simulink model "targeting_subsystem"  (R2020a)
settings: Solver=VariableStepAuto  StartTime=0.0  StopTime=10.0  RelTol=1e-3
settings Model: Creator=Tamer  LastModifiedBy=Tamer

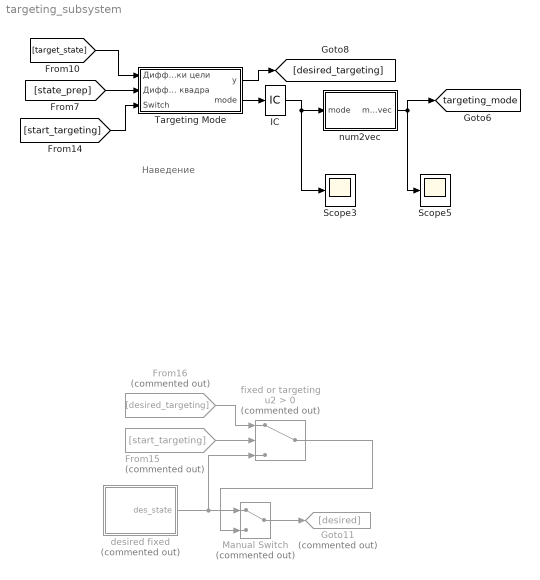
== system targeting_subsystem ==
  note: Наведение
  From15 : From  Commented=on  GotoTag=start_targeting
  From16 : From  Commented=on  GotoTag=desired_targeting
  Goto11 : Goto  Commented=on  GotoTag=desired
  IC : InitialCondition  Value=0
  Manual Switch : ManualSwitch  Commented=on
  Scope3 : Scope
  Scope5 : Scope
  Targeting Mode : Subsystem
  desired fixed : MATLAB Function  Commented=on  TreatAsAtomicUnit=on
  fixed or targeting : Switch  Commented=on  Criteria=u2 > Threshold
  num2vec : MATLAB Function  TreatAsAtomicUnit=on
  tag scope: targeting_mode=global
  wires:
  IC/1 -> num2vec/1(mode), Scope3/1
  num2vec/1(mode_vec) -> [targeting_mode], Scope5/1
  Targeting Mode/1(y) -> [desired_targeting]
  [target_state] -> Targeting Mode/1("Диффурочки цели ")
  Targeting Mode/2(mode) -> IC/1
  [start_targeting] -> Targeting Mode/3(Switch)
  [state_prep] -> Targeting Mode/2(Диффурочки квадра)
  fixed or targeting/1 -> Manual Switch/2
  From15/1 -> fixed or targeting/2
  desired fixed/1(des_state) -> fixed or targeting/3, Manual Switch/1
  From16/1 -> fixed or targeting/1
  Manual Switch/1 -> Goto11/1

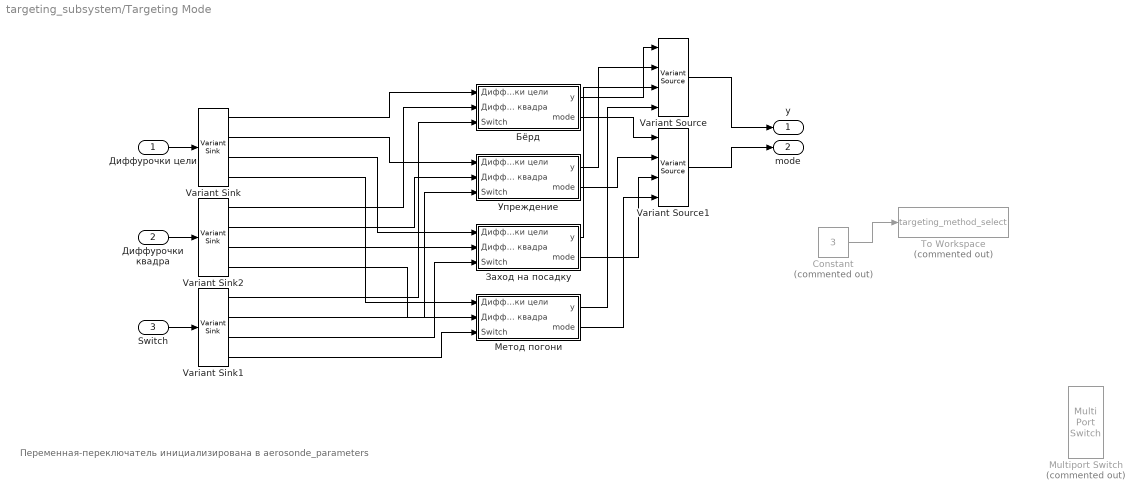
== system targeting_subsystem/Targeting Mode ==
  note: Переменная-переключатель инициализирована в aerosonde_parameters
  "Диффурочки цели " : Inport
  Диффурочки квадра : Inport  Port=2
  Switch : Inport  Port=3
  Constant : Constant  Commented=on  Value=3
  Multiport Switch : MultiPortSwitch  Commented=on  Inputs=4
  To Workspace : ToWorkspace  Commented=on  VariableName=targeting_method_select  SaveFormat=Timeseries  SampleTime=-1
  Variant Sink : VariantSink
  Variant Sink1 : VariantSink
  Variant Sink2 : VariantSink
  Variant Source : VariantSource
  Variant Source1 : VariantSource
  Бёрд : Subsystem
  Заход на посадку : Subsystem
  Метод погони : Subsystem
  Упреждение : Subsystem
  y : Outport
  mode : Outport  Port=2
  wires:
  Упреждение/1(y) -> Variant Source/2
  Упреждение/2(mode) -> Variant Source1/2
  Бёрд/2(mode) -> Variant Source1/1
  Бёрд/1(y) -> Variant Source/1
  Constant/1 -> To Workspace/1
  Заход на посадку/2(mode) -> Variant Source1/3
  Variant Source/1 -> y/1
  Variant Source1/1 -> mode/1
  Метод погони/1(y) -> Variant Source/4
  Метод погони/2(mode) -> Variant Source1/4
  "Диффурочки цели "/1 -> Variant Sink/1
  Диффурочки квадра/1 -> Variant Sink2/1
  Switch/1 -> Variant Sink1/1
  Variant Sink/1 -> Бёрд/1("Диффурочки цели ")
  Variant Sink/2 -> Упреждение/1("Диффурочки цели ")
  Variant Sink/3 -> Заход на посадку/1("Диффурочки цели ")
  Variant Sink/4 -> Метод погони/1("Диффурочки цели ")
  Variant Sink2/1 -> Бёрд/2(Диффурочки квадра)
  Variant Sink2/2 -> Упреждение/2(Диффурочки квадра)
  Variant Sink2/3 -> Заход на посадку/2(Диффурочки квадра)
  Variant Sink2/4 -> Метод погони/2(Диффурочки квадра)
  Variant Sink1/1 -> Бёрд/3(Switch)
  Variant Sink1/2 -> Упреждение/3(Switch)
  Variant Sink1/3 -> Заход на посадку/3(Switch)
  Variant Sink1/4 -> Метод погони/3(Switch)
  Заход на посадку/1(y) -> Variant Source/3

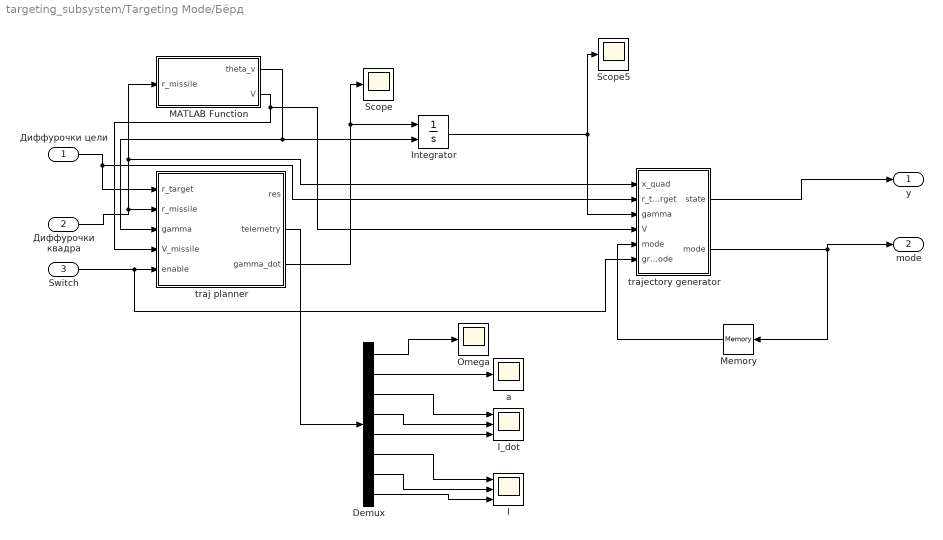
== system targeting_subsystem/Targeting Mode/Бёрд ==
  "Диффурочки цели " : Inport
  Диффурочки квадра : Inport  Port=2
  Switch : Inport  Port=3
  Demux : Demux  Outputs=8
  Integrator : Integrator  InitialConditionSource=external
  MATLAB Function : MATLAB Function  TreatAsAtomicUnit=on
  Memory : Memory
  Omega : Scope
  Scope : Scope
  Scope5 : Scope
  a : Scope
  l : Scope  NumInputPorts=3
  l_dot : Scope  NumInputPorts=3
  traj planner : MATLAB Function  TreatAsAtomicUnit=on
  trajectory generator : MATLAB Function  TreatAsAtomicUnit=on
  y : Outport
  mode : Outport  Port=2
  wires:
  "Диффурочки цели "/1 -> traj planner/1(r_target), trajectory generator/2(r_target)
  trajectory generator/1(state) -> y/1
  Диффурочки квадра/1 -> MATLAB Function/1(r_missile), trajectory generator/1(x_quad), traj planner/2(r_missile)
  MATLAB Function/1(theta_v) -> Integrator/2, traj planner/3(gamma)
  MATLAB Function/2(V) -> traj planner/4(V_missile), trajectory generator/4(V)
  traj planner/3(gamma_dot) -> Scope/1, Integrator/1
  Integrator/1 -> trajectory generator/3(gamma), Scope5/1
  trajectory generator/2(mode) -> mode/1, Memory/1
  Memory/1 -> trajectory generator/5("mode ")
  Switch/1 -> trajectory generator/6(grand_mode), traj planner/5(enable)
  traj planner/2(telemetry) -> Demux/1
  Demux/1 -> Omega/1
  Demux/2 -> a/1
  Demux/3 -> l_dot/1
  Demux/4 -> l_dot/2
  Demux/5 -> l_dot/3
  Demux/6 -> l/1
  Demux/7 -> l/2
  Demux/8 -> l/3

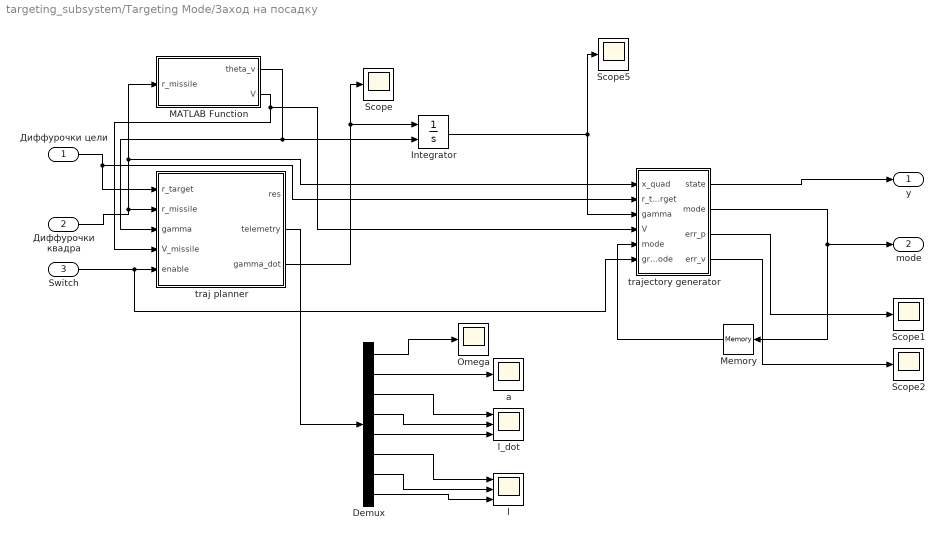
== system targeting_subsystem/Targeting Mode/Заход на посадку ==
  "Диффурочки цели " : Inport
  Диффурочки квадра : Inport  Port=2
  Switch : Inport  Port=3
  Demux : Demux  Outputs=8
  Integrator : Integrator  InitialConditionSource=external
  MATLAB Function : MATLAB Function  TreatAsAtomicUnit=on
  Memory : Memory
  Omega : Scope
  Scope{,1..2,5} (4 alike) : Scope
  a : Scope
  l : Scope  NumInputPorts=3
  l_dot : Scope  NumInputPorts=3
  traj planner : MATLAB Function  TreatAsAtomicUnit=on
  trajectory generator : MATLAB Function  TreatAsAtomicUnit=on
  y : Outport
  mode : Outport  Port=2
  wires:
  "Диффурочки цели "/1 -> traj planner/1(r_target), trajectory generator/2(r_target)
  trajectory generator/1(state) -> y/1
  Диффурочки квадра/1 -> MATLAB Function/1(r_missile), trajectory generator/1(x_quad), traj planner/2(r_missile)
  MATLAB Function/1(theta_v) -> Integrator/2, traj planner/3(gamma)
  MATLAB Function/2(V) -> traj planner/4(V_missile), trajectory generator/4(V)
  traj planner/3(gamma_dot) -> Scope/1, Integrator/1
  Integrator/1 -> trajectory generator/3(gamma), Scope5/1
  trajectory generator/2(mode) -> Memory/1, mode/1
  Memory/1 -> trajectory generator/5("mode ")
  Switch/1 -> trajectory generator/6(grand_mode), traj planner/5(enable)
  traj planner/2(telemetry) -> Demux/1
  Demux/1 -> Omega/1
  Demux/2 -> a/1
  Demux/3 -> l_dot/1
  Demux/4 -> l_dot/2
  Demux/5 -> l_dot/3
  Demux/6 -> l/1
  Demux/7 -> l/2
  Demux/8 -> l/3
  trajectory generator/3(err_p) -> Scope1/1
  trajectory generator/4(err_v) -> Scope2/1

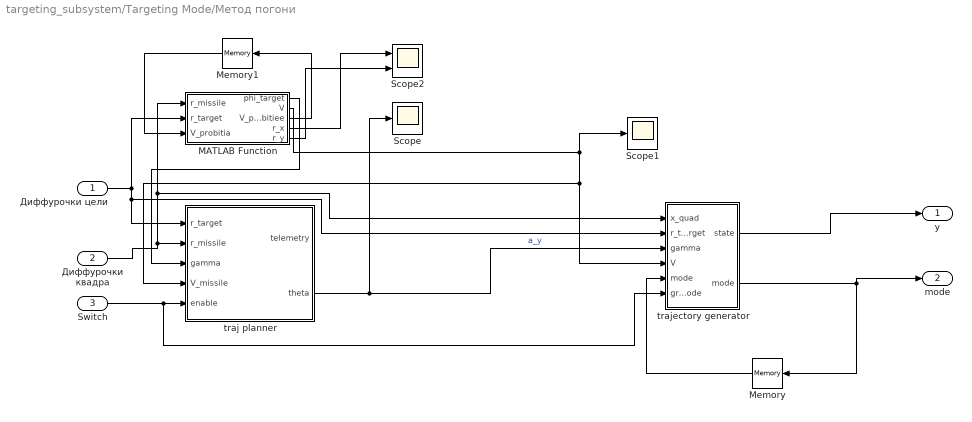
== system targeting_subsystem/Targeting Mode/Метод погони ==
  "Диффурочки цели " : Inport
  Диффурочки квадра : Inport  Port=2
  Switch : Inport  Port=3
  MATLAB Function : MATLAB Function  TreatAsAtomicUnit=on
  Memory : Memory
  Memory1 : Memory
  Scope : Scope
  Scope1 : Scope
  Scope2 : Scope  NumInputPorts=2
  traj planner : MATLAB Function  TreatAsAtomicUnit=on
  trajectory generator : MATLAB Function  TreatAsAtomicUnit=on
  y : Outport
  mode : Outport  Port=2
  wires:
  Memory1/1 -> MATLAB Function/3(V_probitia)
  traj planner/2(theta) -> trajectory generator/3(gamma), Scope/1  "a_y"
  MATLAB Function/2(V) -> Scope1/1, trajectory generator/4(V), traj planner/4(V_missile)
  "Диффурочки цели "/1 -> MATLAB Function/2(r_target), traj planner/1(r_target), trajectory generator/2(r_target)
  MATLAB Function/1(phi_target) -> traj planner/3(gamma)
  Switch/1 -> trajectory generator/6(grand_mode), traj planner/5(enable)
  MATLAB Function/3(V_probitiee) -> Memory1/1
  trajectory generator/2(mode) -> mode/1, Memory/1
  Memory/1 -> trajectory generator/5("mode ")
  Диффурочки квадра/1 -> MATLAB Function/1(r_missile), trajectory generator/1(x_quad), traj planner/2(r_missile)
  trajectory generator/1(state) -> y/1
  MATLAB Function/4(r_x) -> Scope2/1
  MATLAB Function/5(r_y) -> Scope2/2

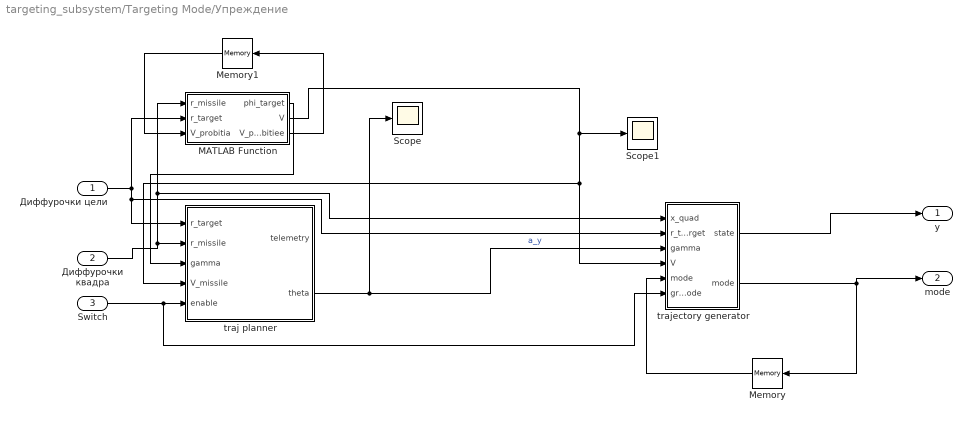
== system targeting_subsystem/Targeting Mode/Упреждение ==
  "Диффурочки цели " : Inport
  Диффурочки квадра : Inport  Port=2
  Switch : Inport  Port=3
  MATLAB Function : MATLAB Function  TreatAsAtomicUnit=on
  Memory : Memory
  Memory1 : Memory
  Scope : Scope
  Scope1 : Scope
  traj planner : MATLAB Function  TreatAsAtomicUnit=on
  trajectory generator : MATLAB Function  TreatAsAtomicUnit=on
  y : Outport
  mode : Outport  Port=2
  wires:
  "Диффурочки цели "/1 -> MATLAB Function/2(r_target), traj planner/1(r_target), trajectory generator/2(r_target)
  trajectory generator/1(state) -> y/1
  Диффурочки квадра/1 -> MATLAB Function/1(r_missile), trajectory generator/1(x_quad), traj planner/2(r_missile)
  MATLAB Function/1(phi_target) -> traj planner/3(gamma)
  trajectory generator/2(mode) -> mode/1, Memory/1
  Memory/1 -> trajectory generator/5("mode ")
  Switch/1 -> trajectory generator/6(grand_mode), traj planner/5(enable)
  traj planner/2(theta) -> trajectory generator/3(gamma), Scope/1  "a_y"
  MATLAB Function/3(V_probitiee) -> Memory1/1
  Memory1/1 -> MATLAB Function/3(V_probitia)
  MATLAB Function/2(V) -> Scope1/1, trajectory generator/4(V), traj planner/4(V_missile)

== matlab function targeting_subsystem/Targeting Mode/Бёрд/traj planner ==
  data: r_target input; res output; r_missile input; gamma input; V_missile input; enable input; telemetry output; gamma_dot output
function [res, telemetry, gamma_dot] = fcn(r_target, r_missile, gamma, V_missile, enable)
[res, telemetry, gamma_dot] = targeting_beard(r_target(1:3), r_target(4:6), r_target(7:9),...
                                            r_missile(1:3), r_missile(4:6), r_missile(10:12), ...
                                            gamma, V_missile, r_missile(8), enable);

== matlab function targeting_subsystem/Targeting Mode/Бёрд/trajectory generator ==
  data: x_quad input; r_target input; gamma input; state output; V input; mode output; mode input; grand_mode input; MAV parameter
function [state, mode] = fcn(x_quad, r_target, gamma, V, mode, grand_mode, MAV)
    state = zeros(3,3);
%     state(:,1) = r_target(1:3);
%     mode = [0; 0];
    
    if grand_mode == 0
        mode = 0;
    else
    if abs(r_target(1) - x_quad(1)) > 3 && abs(r_target(2) - x_quad(2)) > 3 && (mode == 0 || mode == 2)
        mode = 2;
        v_x = V*cos(gamma);
        v_y = V*sin(gamma);
        state(1,2) = v_x;
        state(2,2) = v_y;
    else
        if mode == 5 || (abs(r_target(1) - x_quad(1)) <= 3 && abs(r_target(2) - x_quad(2)) <= 3)
%           стабилизация по обеим осям по координате
            state(1,1) = r_target(1);
            state(2,1) = r_target(2);
            mode = 5;
        else
        v_x = V*cos(gamma);
        v_y = V*sin(gamma);
        if abs(r_target(1) - x_quad(1)) > 3 || mode == 4
%           по У вышли на стабилизацию
            state(1,2) = v_x;
            state(2,1) = r_target(2);
            mode = 4;
        end
        if abs(r_target(2) - x_quad(2)) > 3 || mode == 3
%           по X вышли на стабилизацию
            state(2,2) = v_y;
            state(1,1) = r_target(1);
            if mode == 4
                mode = 5;
            else
                mode = 3;
            end
        end
        end
%         if mode == 5 || flag == 1
% %           стабилизация по обеим осям
%             state(1,1) = r_target(1);
%             state(2,1) = r_target(2);
%             state(1,2) = 0;
%             state(2,2) = 0;
%             mode = 5;
%         end
    end
    end

== matlab function targeting_subsystem/Targeting Mode/Упреждение/MATLAB Function ==
  data: r_missile input; phi_target output; V output; r_target input; V_probitia input; V_probitiee output
function [phi_target, V, V_probitiee] = fcn(r_missile, r_target, V_probitia)

    r_x = r_target(1) - r_missile(1);
    r_y = r_target(2) - r_missile(2);
    
    phi_target = atan2(r_y, r_x);
    
    V = 10; 
    l = sqrt(r_x^2 + r_y^2);
    L_treshold = 10;
%     if l < L_treshold
%         if V_probitia == 0
%             vx = r_missile(4);
%             vy = r_missile(5);
%             V_probitia = sqrt(vx.^2 + vy.^2);
%         end
%         V = max(10*(l/L_treshold), 2)
%     end
    V_probitiee = V_probitia;

== matlab function targeting_subsystem/Targeting Mode/Метод погони/trajectory generator ==
  data: x_quad input; r_target input; gamma input; state output; V input; mode output; mode input; grand_mode input; MAV parameter
function [state, mode] = fcn(x_quad, r_target, gamma, V, mode, grand_mode, MAV)
    state = zeros(3,3);
%     state(:,1) = r_target(1:3);
%     mode = [0; 0];

    
    
    if grand_mode == 0
        mode = 0;
    else
    if abs(r_target(1) - x_quad(1)) > 3 && abs(r_target(2) - x_quad(2)) > 3 && (mode == 0 || mode == 2)
        mode = 2;
        v_x = V*cos(gamma);
        v_y = V*sin(gamma);
        state(1,2) = v_x;
        state(2,2) = v_y;
    else
        if mode == 5 || (abs(r_target(1) - x_quad(1)) <= 3 && abs(r_target(2) - x_quad(2)) <= 3)
%           стабилизация по обеим осям по координате
        state(1,1) = r_target(1);
        state(2,1) = r_target(2);
        mode = 5;
        else
        v_x = V*cos(gamma);
        v_y = V*sin(gamma);
        if abs(r_target(1) - x_quad(1)) > 3 || mode == 4
    %           по У вышли на стабилизацию
            state(1,2) = v_x;
            state(2,1) = r_target(2);
            if mode == 3
                mode = 5;
            else
                mode = 4;
            end
        end
        if abs(r_target(2) - x_quad(2)) > 3 || mode == 3
    %           по X вышли на стабилизацию
            state(2,2) = v_y;
            state(1,1) = r_target(1);
            if mode == 4
                mode = 5;
            else
                mode = 3;
            end
        end
        end
    end
    end

== matlab function targeting_subsystem/Targeting Mode/Упреждение/traj planner ==
  data: telemetry output; r_target input; theta output; r_missile input; gamma input; V_missile input; enable input
function [ telemetry, theta] = fcn(r_target, r_missile, gamma, V_missile, enable)
[telemetry, theta] = targeting_forestalling(r_target(1:3), r_target(4:6), r_target(7:9),...
                                            r_missile(1:3), r_missile(4:6), r_missile(10:12), ...
                                            gamma, V_missile, r_missile(8), enable, deg2rad(10));

== matlab function targeting_subsystem/Targeting Mode/Упреждение/trajectory generator ==
  data: x_quad input; r_target input; gamma input; state output; V input; mode output; mode input; grand_mode input; MAV parameter
function [state, mode] = fcn(x_quad, r_target, gamma, V, mode, grand_mode, MAV)
    state = zeros(3,3);
%     state(:,1) = r_target(1:3);
%     mode = [0; 0];

    
    
    if grand_mode == 0
        mode = 0;
    else
    if abs(r_target(1) - x_quad(1)) > 3 && abs(r_target(2) - x_quad(2)) > 3 && (mode == 0 || mode == 2)
        mode = 2;
        v_x = V*cos(gamma);
        v_y = V*sin(gamma);
        state(1,2) = v_x;
        state(2,2) = v_y;
    else
        if mode == 5 || (abs(r_target(1) - x_quad(1)) <= 3 && abs(r_target(2) - x_quad(2)) <= 3)
%           стабилизация по обеим осям по координате
        state(1,1) = r_target(1);
        state(2,1) = r_target(2);
        mode = 5;
        else
        v_x = V*cos(gamma);
        v_y = V*sin(gamma);
        if abs(r_target(1) - x_quad(1)) > 3 || mode == 4
    %           по У вышли на стабилизацию
            state(1,2) = v_x;
            state(2,1) = r_target(2);
            if mode == 3
                mode = 5;
            else
                mode = 4;
            end
        end
        if abs(r_target(2) - x_quad(2)) > 3 || mode == 3
    %           по X вышли на стабилизацию
            state(2,2) = v_y;
            state(1,1) = r_target(1);
            if mode == 4
                mode = 5;
            else
                mode = 3;
            end
        end
        end
    end
    end

== matlab function targeting_subsystem/num2vec ==
  data: mode input; mode_vec output
function mode_vec = fcn(mode)
mode_vec = [0 0]';
switch round(mode)
    case 0
        mode_vec = [0 0]';
    case 2
        mode_vec = [1 1]';
    case 3
        mode_vec = [2 1]';
    case 4
        mode_vec = [1 2]';
    case 5
        mode_vec = [2 2]';
    case 6
        mode_vec = [2 3]';
    case 7
        mode_vec = [-1 -1]';
    otherwise
        mode_vec = [0 0]';
end
% mode_vec = mode_vec';

== matlab function targeting_subsystem/desired fixed ==
  data: des_state output; MAV parameter
function des_state = fcn(  MAV)

% pos = [90.0000  9.3678 0]';
pos = [MAV.x0  MAV.y0 MAV.z0]';
vel = [0 0 0]';
acc = [0 0 0]';
des_state = [pos vel acc];

== matlab function targeting_subsystem/Targeting Mode/Заход на посадку/MATLAB Function ==
  data: r_missile input; theta_v output; V output
function [theta_v, V] = fcn(r_missile)
%   скорости ракеты в земной СК
    vx = r_missile(4);
    vy = r_missile(5);
    vz = r_missile(6);

    theta_v = atan2(vy, vx);
    V = sqrt(vx.^2 + vy.^2 + vz.^2);
    
    V = 10;

== matlab function targeting_subsystem/Targeting Mode/Метод погони/MATLAB Function ==
  data: r_missile input; phi_target output; V output; r_target input; V_probitia input; V_probitiee output; r_x output; r_y output
function [phi_target, V, V_probitiee, r_x, r_y] = fcn(r_missile, r_target, V_probitia)

    r_x = r_target(1) - r_missile(1);
    r_y = r_target(2) - r_missile(2);
    
    phi_target = atan2(r_y, r_x);
    
    V = 10; 
%     l = sqrt(r_x^2 + r_y^2);
%     L_treshold = 10;
%     if l < L_treshold
%         if V_probitia == 0
%             vx = r_missile(4);
%             vy = r_missile(5);
%             V_probitia = sqrt(vx.^2 + vy.^2);
%         end
%         V = max(10*(l/L_treshold), 2)
%     end
    V_probitiee = V_probitia;

== matlab function targeting_subsystem/Targeting Mode/Заход на посадку/traj planner ==
  data: r_target input; res output; r_missile input; gamma input; V_missile input; enable input; telemetry output; gamma_dot output
function [res, telemetry, gamma_dot] = fcn(r_target, r_missile, gamma, V_missile, enable)

r_target(2) = r_target(2) + 1;

[res, telemetry, gamma_dot] = targeting_beard(r_target(1:3), r_target(4:6), r_target(7:9),...
                                            r_missile(1:3), r_missile(4:6), r_missile(10:12), ...
                                            gamma, V_missile, r_missile(8), enable);

== matlab function targeting_subsystem/Targeting Mode/Заход на посадку/trajectory generator ==
  data: x_quad input; r_target input; gamma input; state output; V input; mode output; mode input; grand_mode input; MAV parameter; err_p output; err_v output
function [state, mode, err_p, err_v] = fcn(x_quad, r_target, gamma, V, mode, grand_mode, MAV)
    state = zeros(3,3);
%     state(:,1) = r_target(1:3);
%     mode = [0; 0];
    err_p = zeros(3,1);
    err_v = zeros(3,1);
    
    if grand_mode == 0
        mode = 0;
    else
        if mode <= 5
            [mode, state] = beard_flight(x_quad, r_target, gamma, V, mode, state);
        end
%         if abs(r_target(1) - x_quad(1)) > 3 && abs(r_target(2) - x_quad(2)) > 3 && (mode == 0 || mode == 2)
%             mode = 2;
%             v_x = V*cos(gamma);
%             v_y = V*sin(gamma);
%             state(1,2) = v_x;
%             state(2,2) = v_y;
%         else
%             r_target_meth2 = r_target(:,:);
%             r_target_meth2(2) = r_target_meth2(2) + 1;  % по этому методу целимся на метр выше в режиме быстрой стабилизации
%             if mode == 5 || (abs(r_target_meth2(1) - x_quad(1)) <= 3 && abs(r_target_meth2(2) - x_quad(2)) <= 3)
%     %           стабилизация по обеим осям по координате
%                 state(1,1) = r_target_meth2(1);
%                 state(2,1) = r_target_meth2(2);
%                 mode = 5;
%             else
%             v_x = V*cos(gamma);
%             v_y = V*sin(gamma);
%             if abs(r_target_meth2(1) - x_quad(1)) > 3 || mode == 4
%     %           по У вышли на стабилизацию
%                 state(1,2) = v_x;
%                 state(2,1) = r_target_meth2(2);
%                 mode = 4;
%             end
%             if abs(r_target_meth2(2) - x_quad(2)) > 3 || mode == 3
%     %           по X вышли на стабилизацию
%                 state(2,2) = v_y;
%                 state(1,1) = r_target_meth2(1);
%                 if mode == 4
%                     mode = 5;
%                 else
%                     mode = 3;
%                 end
%             end
%             end
%         end
        err_p = r_target(1:3) - x_quad(1:3);
        err_v = r_target(4:6) - x_quad(4:6);
        if sum(abs(err_p + [0 1 0]')) < 0.5 && sum(abs(err_v)) < 0.5 || mode == 6 || mode == 7
            state = zeros(3,3);
            state(1,1) = r_target(1);
%             state(1,2) = r_target(4);
            state(2,2) = MAV.Modes.Soft_falling_1.Falling_speed + r_target(5);
            if abs(err_p(2)) < 0.02 || mode == 7
                mode = 7;
            else
               mode = 6;
            end
        end
    end
    
function [mode, state] = beard_flight(x_quad, r_target, gamma, V, mode, state)
if abs(r_target(1) - x_quad(1)) > 3 && abs(r_target(2) - x_quad(2)) > 3 && (mode == 0 || mode == 2)
    mode = 2;
    v_x = V*cos(gamma);
    v_y = V*sin(gamma);
    state(1,2) = v_x;
    state(2,2) = v_y;
else
    r_target_meth2 = r_target(:,:);
    r_target_meth2(2) = r_target_meth2(2) + 1;  % по этому методу целимся на метр выше в режиме быстрой стабилизации
    if mode == 5 || (abs(r_target_meth2(1) - x_quad(1)) <= 2.5 && abs(r_target_meth2(2) - x_quad(2)) <= 3)
%           стабилизация по обеим осям по координате
        state(1,1) = r_target_meth2(1);
        state(2,1) = r_target_meth2(2);
        mode = 5;
    else
    v_x = V*cos(gamma);
    v_y = V*sin(gamma);
    if abs(r_target_meth2(1) - x_quad(1)) > 2.5 || mode == 4
%           по У вышли на стабилизацию
        state(1,2) = v_x;
        state(2,1) = r_target_meth2(2);
        mode = 4;
    end
    if abs(r_target_meth2(2) - x_quad(2)) > 3 || mode == 3
%           по X вышли на стабилизацию
        state(2,2) = v_y;
        state(1,1) = r_target_meth2(1);
        if mode == 4
            mode = 5;
        else
            mode = 3;
        end
    end
    end
end

== matlab function targeting_subsystem/Targeting Mode/Бёрд/MATLAB Function ==
  data: r_missile input; theta_v output; V output
function [theta_v, V] = fcn(r_missile)
%   скорости ракеты в земной СК
    vx = r_missile(4);
    vy = r_missile(5);
    vz = r_missile(6);

    theta_v = atan2(vy, vx);
    V = sqrt(vx.^2 + vy.^2 + vz.^2);
    
    V = 10;

== matlab function targeting_subsystem/Targeting Mode/Метод погони/traj planner ==
  data: telemetry output; r_target input; theta output; r_missile input; gamma input; V_missile input; enable input
function [ telemetry, theta] = fcn(r_target, r_missile, gamma, V_missile, enable)
[telemetry, theta] = targeting_forestalling(r_target(1:3), r_target(4:6), r_target(7:9),...
                                            r_missile(1:3), r_missile(4:6), r_missile(10:12), ...
                                            gamma, V_missile, r_missile(8), enable, 0);
